simulink model "simulacao_motor_sincrono"  (R2016a)
settings: Solver=FixedStepDiscrete  StartTime=0.0  StopTime=12  RelTol=1e-3
PreLoadFcn:
  | Ts=2e-6;
libraries: powerlib x2, powerlib_meascontrol x2, electricdrivelib x1
Description:
  | Copyright 2008-2016 The MathWorks, Inc.
settings Model: ExtModeAutoUpdateStatusClock=off  Creator=MathWorks  LastModifiedBy=fikch
settings DataIOCC: LimitDataPoints=on  SaveFormat=Array  SignalLoggingSaveFormat=ModelDataLogs  SaveOutput=off  SignalLogging=off  SaveTime=off  SignalLoggingName=sigsOut
settings OptimizationCC: ExpressionDepthLimit=2147483647  InitFltsAndDblsToZero=on
settings DebuggingCC: UnderspecifiedInitializationDetection=Classic  MergeDetectMultiDrivingBlocksExec=none  CheckExecutionContextPreStartOutputMsg=on  CheckExecutionContextRuntimeOutputMsg=on  SignalResolutionControl=TryResolveAllWithWarning  MultiTaskDSMMsg=warning  MultiTaskCondExecSysMsg=none  FcnCallInpInsideContextMsg=UseLocalSettings  StateNameClashWarn=warning
settings HardwareCC: ProdBitPerPointer=32  ProdLargestAtomicFloat=None  ProdIntDivRoundTo=Undefined  ProdEndianess=Unspecified  ProdWordSize=32  ProdHWDeviceType=32-bit Generic  TargetUnknown=on
settings ModelReferenceCC: PropagateSignalLabelsOutOfModel=off
settings GRTTargetCC: CombineOutputUpdateFcns=off  GRTInterface=on
settings ConfigComp: CovModelRefEnable=Off  CovSFcnEnable=off

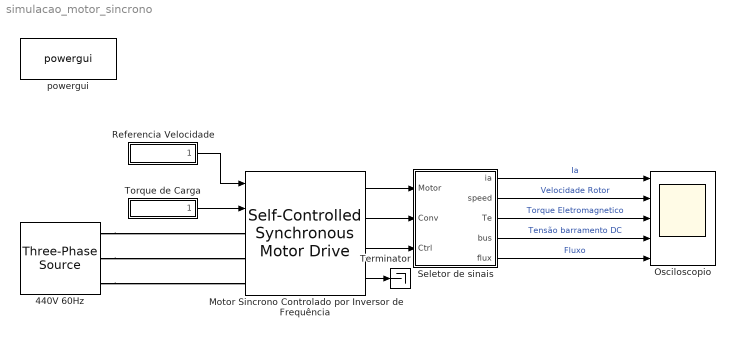
== system simulacao_motor_sincrono ==
  440V 60Hz : powerlib/Electrical Sources/Three-Phase Source  InternalConnection=Yg  VoltagePhases=off  Voltage=440  PhaseAngle=0  Voltage_phases=[25e3 25e3 25e3]/sqrt(3)  PhaseAngles_phases=[0 -120 +120]  Frequency=60  NonIdealSource=on  SpecifyImpedance=off  Resistance=0.02  Inductance=0.05e-3  ShortCircuitLevel=100e6  BaseVoltage=25e3  XRratio=7  BusType=swing  Pref=0  Qref=0  Prefabc=[10e3, 10e3, 10e3]  Qrefabc=[0, 0, 0]  Qmin=-inf  Qmax=inf
  Motor Sincrono Controlado por Inversor de Frequência : electricdrivelib/AC drives/Self-Controlled Synchronous Motor Drive  showMaskWarnings=on  AverageValue=off  MechanicalLoad=Torque Tm  driveType=AC5  outputBusMode=Multiple output buses  baseSampleTime=2e-06
      link override Vector control: kpfl=2000  kifl=10000  flc_lpf=100  flc_sat=[-400,400]  mag_hvt=0  mag_v=0  mag_tot=0.5  fnv=73.4  h=1  Tvect=20e-6  Rs=1.62  p=2  daf=5
  Osciloscopio : Scope  NumInputPorts=5
  Referencia Velocidade : Subsystem
  Seletor de sinais : Subsystem
  Terminator : Terminator
  Torque de Carga : Subsystem
  powergui : powerlib/powergui  Priority=2  SimulationMode=Discrete  SolverType=Tustin/Backward Euler (TBE)  SampleTime=Ts  frequency=60  SPID=off  DisableSnubberDevices=off  DisableRonSwitches=off  DisableVfSwitches=off  SwTol=0  DisplayEquations=off  Interpol=off  ExternalGateDelay=off  methode=off  Ts=0  FunctionMessages=off  echomessages=off  HookPort=off  EnableUseOfTLC=off  x0status=blocks  frequencyindice=60  Pbase=100e6  ErrMax=1e-4  Iterations=50  UnitsV=kV  UnitsW=MW  buscounter=0  RestoreLinks=warning  ResistiveCurrentMeasurement=off  Frange=[0:2:500]  Ylog=off  Xlog=on  ShowGrid=off  save=off  variable=ZData  structure=0  ZoomFFT=on  StartTime=0.0  cycles=1  DisplayStyle=1  fundamental=60  FreqAxis=off  MaxFrequency=1000  frequencyindicesteady=1  RmsSteady=1  display=off
  wires:
  Motor Sincrono Controlado por Inversor de Frequência/1 -> Seletor de sinais/1(Motor)
  Motor Sincrono Controlado por Inversor de Frequência/2 -> Seletor de sinais/2(Conv)
  Motor Sincrono Controlado por Inversor de Frequência/3 -> Seletor de sinais/3(Ctrl)
  Torque de Carga/1(" ") -> Motor Sincrono Controlado por Inversor de Frequência/2
  Referencia Velocidade/1(" ") -> Motor Sincrono Controlado por Inversor de Frequência/1
  Seletor de sinais/1(ia) -> Osciloscopio/1  "Ia"
  Seletor de sinais/2(speed) -> Osciloscopio/2  "Velocidade Rotor"
  Seletor de sinais/3(Te) -> Osciloscopio/3  "Torque Eletromagnetico"
  Seletor de sinais/4(bus) -> Osciloscopio/4  "Tensão barramento DC"
  Seletor de sinais/5(flux) -> Osciloscopio/5  "Fluxo"
  Motor Sincrono Controlado por Inversor de Frequência/4 -> Terminator/1
  connections:
  440V 60Hz/RConn1 -- Motor Sincrono Controlado por Inversor de Frequência/LConn1
  440V 60Hz/RConn2 -- Motor Sincrono Controlado por Inversor de Frequência/LConn2
  440V 60Hz/RConn3 -- Motor Sincrono Controlado por Inversor de Frequência/LConn3

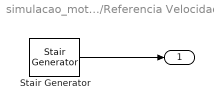
== system simulacao_motor_sincrono/Referencia Velocidade ==
  Stair Generator : powerlib_meascontrol/Pulse & Signal Generators/Stair Generator  t=[1 9]  e=[188.5 0]  Ts=Ts
  " " : Outport
  wires:
  Stair Generator/1 -> " "/1

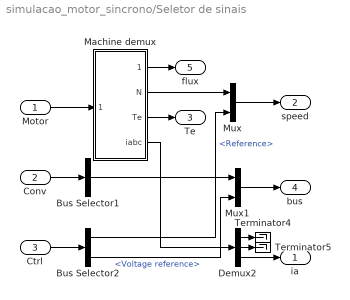
== system simulacao_motor_sincrono/Seletor de sinais ==
  Motor : Inport
  Conv : Inport  Port=2
  Ctrl : Inport  Port=3
  Bus Selector1 : BusSelector  OutputSignals=V bus (V)  OutputAsBus=on
  Bus Selector2 : BusSelector  OutputSignals=Speed&Torque controller.Reference,Active Rectifier.Voltage reference
  Demux2 : Demux  Outputs=3
  Machine demux : Subsystem
  Mux : Mux  Inputs=2
  Mux1 : Mux  Inputs=2
  Terminator4 : Terminator
  Terminator5 : Terminator
  ia : Outport
  speed : Outport  Port=2
  Te : Outport  Port=3
  bus : Outport  Port=4
  flux : Outport  Port=5
  wires:
  Ctrl/1 -> Bus Selector2/1
  Machine demux/2(N) -> Mux/1
  Mux/1 -> speed/1
  Demux2/1 -> Terminator4/1
  Demux2/2 -> Terminator5/1
  Demux2/3 -> ia/1
  Machine demux/4(iabc) -> Demux2/1
  Machine demux/3("Te ") -> Te/1
  Machine demux/1(|flux|) -> flux/1
  Mux1/1 -> bus/1
  Conv/1 -> Bus Selector1/1
  Bus Selector1/1 -> Mux1/1
  Motor/1 -> Machine demux/1(m_SI)
  Bus Selector2/2 -> Mux1/2  "<Voltage reference>"
  Bus Selector2/1 -> Mux/2  "<Reference>"

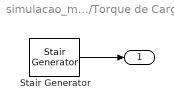
== system simulacao_motor_sincrono/Torque de Carga ==
  Stair Generator : powerlib_meascontrol/Pulse & Signal Generators/Stair Generator  t=[4 7 ]  e=[-7 0 ]  Ts=Ts
  " " : Outport
  wires:
  Stair Generator/1 -> " "/1

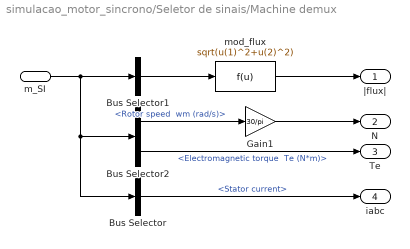
== system simulacao_motor_sincrono/Seletor de sinais/Machine demux ==
  m_SI : Inport
  Bus Selector : BusSelector  OutputSignals=Stator current
  Bus Selector1 : BusSelector  OutputSignals="dq0 components.Mutual flux  phimq (V s),dq0 components.Mutual flux  phimd (V s)"  OutputAsBus=on
  Bus Selector2 : BusSelector  OutputSignals="Mechanical.Rotor speed  wm (rad/s),Mechanical.Electromagnetic torque  Te (N*m)"
  Gain1 : Gain  Gain=30/pi  SaturateOnIntegerOverflow=on  OutDataTypeStr=Inherit: Same as input  ParamDataTypeStr=Inherit: Same as input
  mod_flux : Fcn  Expr=sqrt(u(1)^2+u(2)^2)
  |flux| : Outport
  N : Outport  Port=2
  "Te " : Outport  Port=3
  iabc : Outport  Port=4
  wires:
  m_SI/1 -> Bus Selector1/1, Bus Selector2/1, Bus Selector/1
  mod_flux/1 -> |flux|/1
  Gain1/1 -> N/1
  Bus Selector/1 -> iabc/1  "<Stator current>"
  Bus Selector1/1 -> mod_flux/1
  Bus Selector2/1 -> Gain1/1  "<Rotor speed  wm (rad/s)>"
  Bus Selector2/2 -> "Te "/1  "<Electromagnetic torque  Te (N*m)>"
